simulink model "WR_Control_LQR"  (R2019a)
settings: Solver=VariableStepAuto  StartTime=0.0  StopTime=10  RelTol=1e-6
values from neighbouring files (symbols this model uses):
  KK7 = lqr(A,B,Q,R)    [thongsoxe2banh.m]
settings Model: Creator=phuon  LastModifiedBy=Duong
settings DataIOCC: ReturnWorkspaceOutputs=off
settings DebuggingCC: ArithmeticOperatorsInVariantConditions=warning
settings SFSimCC: SimUseLocalCustomCode=off
settings RTWCC: RTWUseLocalCustomCode=off

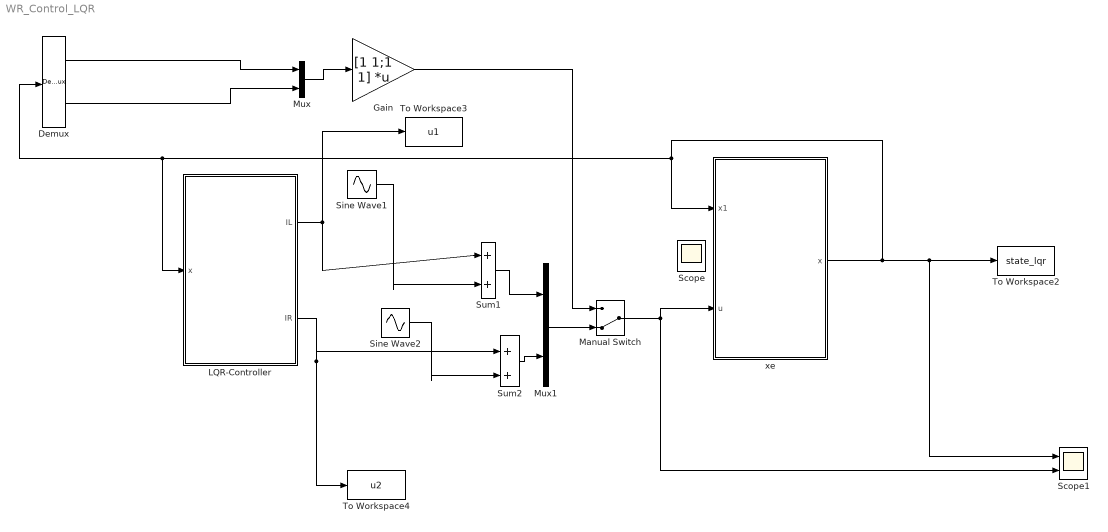
== system WR_Control_LQR ==
  Demux : Demux  Outputs=6
  Gain : Gain  Gain=[1 1;1 1]  Multiplication=Matrix(K*u)
  LQR-Controller : Subsystem
  Manual Switch : ManualSwitch  CurrentSetting=0
  Mux : Mux  Inputs=2
  Mux1 : Mux  Inputs=2
  Scope : Scope
  Scope1 : Scope  NumInputPorts=2
  Sine Wave1 : Sin  Amplitude=0  Bias=.2  Phase=pi/6  SampleTime=0
  Sine Wave2 : Sin  Amplitude=0  Bias=-.2  Frequency=2  Phase=pi/4  SampleTime=0
  Sum1 : Sum  Inputs=|++
  Sum2 : Sum  Inputs=|++
  To Workspace2 : ToWorkspace  VariableName=state_lqr  SaveFormat=Timeseries  SampleTime=-1
  To Workspace3 : ToWorkspace  VariableName=u1  SaveFormat=Timeseries  SampleTime=-1
  To Workspace4 : ToWorkspace  VariableName=u2  SaveFormat=Timeseries  SampleTime=-1
  "xe " : Subsystem
  wires:
  "xe "/1(x) -> Scope1/1, To Workspace2/1, Demux/1, LQR-Controller/1(x), "xe "/1(x1)
  LQR-Controller/2(IR) -> To Workspace4/1, Sum2/1
  LQR-Controller/1(IL) -> Sum1/1, To Workspace3/1
  Sine Wave1/1 -> Sum1/2
  Sum1/1 -> Mux1/1
  Sine Wave2/1 -> Sum2/2
  Sum2/1 -> Mux1/2
  Demux/2 -> Mux/1
  Demux/5 -> Mux/2
  Mux/1 -> Gain/1
  Gain/1 -> Manual Switch/1
  Manual Switch/1 -> Scope1/2, "xe "/2(u)
  Mux1/1 -> Manual Switch/2

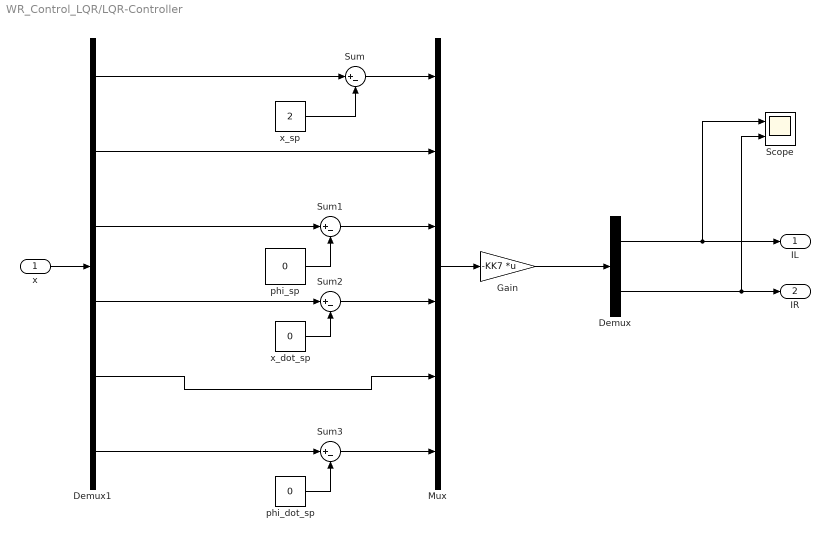
== system WR_Control_LQR/LQR-Controller ==
  x : Inport
  Demux : Demux  Outputs=2
  Demux1 : Demux  Outputs=6
  Gain : Gain  Gain=-KK7  Multiplication=Matrix(K*u)
  Mux : Mux  Inputs=6
  Scope : Scope  NumInputPorts=2
  Sum{,1..3} (4 alike) : Sum  Inputs=|+-
  "phi_dot_sp " : Constant  Value=0
  "phi_sp " : Constant  Value=0
  "x_dot_sp " : Constant  Value=0
  "x_sp " : Constant  Value=2
  IL : Outport
  IR : Outport  Port=2
  wires:
  Sum/1 -> Mux/1
  Demux1/1 -> Sum/1
  Demux1/2 -> Mux/2
  Sum1/1 -> Mux/3
  Demux1/3 -> Sum1/1
  "phi_sp "/1 -> Sum1/2
  Sum2/1 -> Mux/4
  Demux1/4 -> Sum2/1
  "x_dot_sp "/1 -> Sum2/2
  Demux1/6 -> Sum3/1
  "phi_dot_sp "/1 -> Sum3/2
  Sum3/1 -> Mux/6
  Demux1/5 -> Mux/5
  Mux/1 -> Gain/1
  Gain/1 -> Demux/1
  Demux/2 -> Scope/2, IR/1
  Demux/1 -> Scope/1, IL/1
  "x_sp "/1 -> Sum/2
  x/1 -> Demux1/1

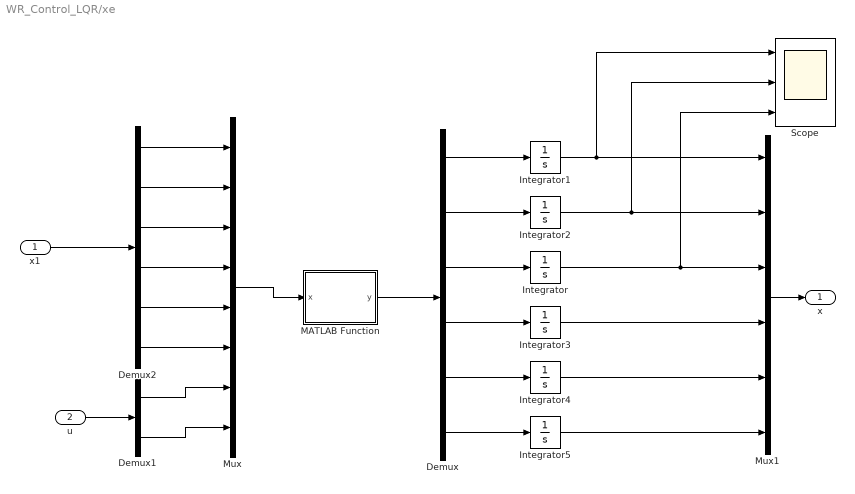
== system WR_Control_LQR/xe  ==
  x1 : Inport
  u : Inport  Port=2
  Demux : Demux  Outputs=6
  Demux1 : Demux  Outputs=2
  Demux2 : Demux  Outputs=6
  Integrator{,1,3..5} (5 alike) : Integrator
  Integrator2 : Integrator  InitialCondition=0.6
  MATLAB Function : MATLAB Function  TreatAsAtomicUnit=on
  Mux : Mux  Inputs=8
  Mux1 : Mux  Inputs=6
  Scope : Scope  NumInputPorts=3
  x : Outport
  wires:
  Demux/2 -> Integrator2/1
  Demux/3 -> Integrator/1
  Demux/6 -> Integrator5/1
  Demux/1 -> Integrator1/1
  Mux/1 -> MATLAB Function/1(x)
  MATLAB Function/1(y) -> Demux/1
  Demux/4 -> Integrator3/1
  Demux/5 -> Integrator4/1
  Demux1/1 -> Mux/7
  Demux1/2 -> Mux/8
  u/1 -> Demux1/1
  Integrator1/1 -> Scope/1, Mux1/1
  Integrator2/1 -> Scope/2, Mux1/2
  Integrator/1 -> Mux1/3, Scope/3
  Integrator3/1 -> Mux1/4
  Integrator4/1 -> Mux1/5
  Integrator5/1 -> Mux1/6
  Mux1/1 -> x/1
  x1/1 -> Demux2/1
  Demux2/6 -> Mux/6
  Demux2/5 -> Mux/5
  Demux2/3 -> Mux/3
  Demux2/4 -> Mux/4
  Demux2/2 -> Mux/2
  Demux2/1 -> Mux/1

== matlab function WR_Control_LQR/xe /MATLAB Function ==
  data: x input; y output
function y = fcn(x)
y = zeros(6,1);
M = 0.765;
m = 0.03;
l = 0.10;
d =0.195;
r = 0.033;

I2 = M*l^2/2; %Momen quan tinh cua than xe doi voi goc theta
I3 = M*(d^2)/2; %Momen quan tinh cua than xe doi voi goc phi
I1 = I3;

J = m*r^2/2; %Momen quan tinh cua banh xe theo truc cua banh
K = m*r^2/4; %Momen quan tinh cua banh xe voi truc thang dung

g = 9.81;
C = 0.005;
x1 = x(1);
x2 = x(2);
x3 = x(3);
x4 = x(4); 
x5 = x(5);
x6 = x(6);
u1 = x(7);
u2 = x(8);
O1 = r^2*(M*l^2+I2)*((u1+u2)/r+2*C*(x5-x4/r)/r+M*l*sin(x2)*(x5^2+x6^2));
O2 = r^2*M*l*cos(x2)*(cos(x2)*sin(x2)*(I3-M*l^2-I1)*x6^2+(u1+u2)+2*C*(x5-x4/r)-M*l*g*sin(x2));
O3 = (2*J+(M+2*m)*r^2)*(cos(x2)*sin(x2)*(M*l^2+I1-I3)*x6^2-(u1+u2)-2*C*(x5-x4/r)+M*l*g*sin(x2));
O4 = -M*l*r^2*cos(x2)*((u1+u2)/r+2*C*(x5-x4/r)/r+M*l*sin(x2)*(x5^2+x6^2));
O5 = -2*r^2*(d*(u1-u2)/(2*r)+x6*sin(x2)*(M*l*x4+2*x5*cos(x2)*(M*l^2+I1-I3))+C*d^2*x6/(2*r^2));
O6 = r^2*(2*I3+4*K+m*d^2+2*(M*l^2+I1-I3)*(sin(x2))^2)+J*d^2;
O = (M*l*r)^2*(1-(cos(x2))^2)+2*I2*J+2*J*M*l^2+(I2*M+2*I2*m+2*M*m*l^2)*r^2;
y = [x4 x5 x6 (O1+O2)/O (O3+O4)/O O5/O6]';
end
